simulink model "bpsk_class"  (R2018a)
settings: Solver=VariableStepAuto  StartTime=0.0  StopTime=8  RelTol=1e-3
libraries: commrandsrc3 x1, dsparch4 x1
settings Model: Creator=hp  LastModifiedBy=hp

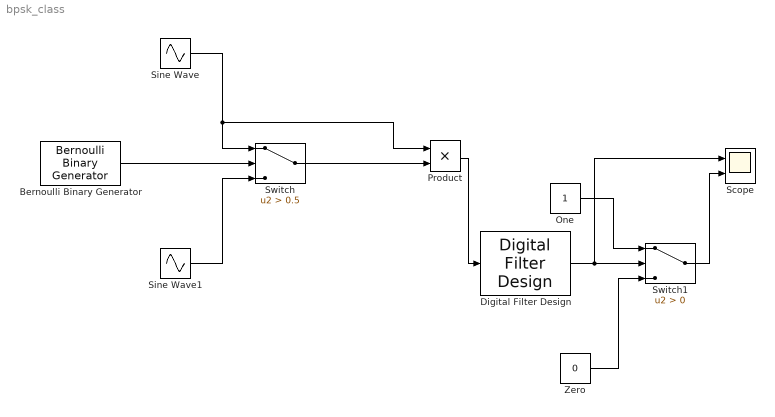
== system bpsk_class ==
  Bernoulli Binary Generator : commrandsrc3/Bernoulli Binary Generator  ProbabilityOfZero=0.5  SeedSource=Parameter  Seed=10  SampleTime=1  SamplesPerFrame=1  OutputDataType=double  SimulateUsing=Interpreted execution
  Digital Filter Design : dsparch4/Digital Filter Design  mwdsp_browser_bugfix_var=off
  One : Constant
  Product : Product
  Scope : Scope  NumInputPorts=2
  Sine Wave : Sin  Frequency=2*pi*1  SampleTime=0.0001
  Sine Wave1 : Sin  Frequency=2*pi*1  Phase=180  SampleTime=0.0001
  Switch : Switch  Criteria=u2 > Threshold  Threshold=0.5
  Switch1 : Switch  Criteria=u2 > Threshold
  Zero : Constant  Value=0
  wires:
  Bernoulli Binary Generator/1 -> Switch/2
  Sine Wave1/1 -> Switch/3
  Switch/1 -> Product/2
  Sine Wave/1 -> Product/1, Switch/1
  Product/1 -> Digital Filter Design/1
  Digital Filter Design/1 -> Scope/1, Switch1/2
  Switch1/1 -> Scope/2
  One/1 -> Switch1/1
  Zero/1 -> Switch1/3
